simulink subsystem "Find_U_And_Powers"  (R2023b)
settings: Solver=VariableStepAuto  StartTime=0.0  StopTime=10.0  RelTol=1e-3
undefined symbols (not defined in the file): Spline_Num_Samples
settings Model: Creator=FIRSTMentor  LastModifiedBy=FIRSTMentor

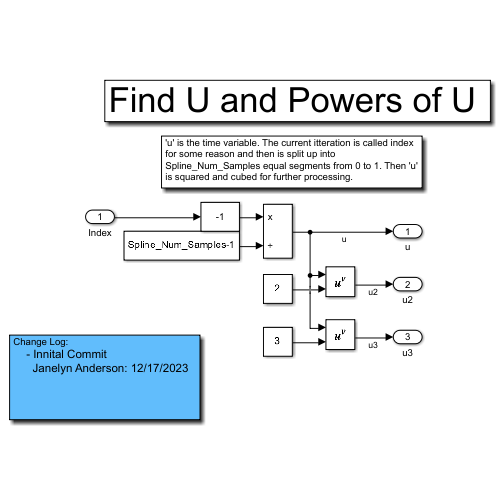
[thumbnail: Simulink's stored preview of the top-level diagram]
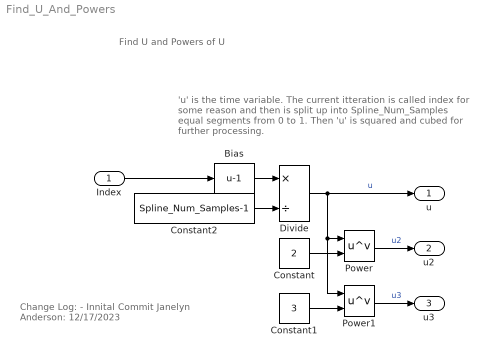
== system Find_U_And_Powers ==
  note: Change Log:
      | - Innital Commit
      | Janelyn Anderson: 12/17/2023
  note: Find U and Powers of U
  note: 'u' is the time variable. The current itteration is called index for some reason and then is split up into Spline_Num_Samples equal segments from 0 to 1. Then 'u' is squared and cubed for further processing.
  Index : Inport
  Bias : Bias  Bias=-1  SaturateOnIntegerOverflow=off
  Constant : Constant  Value=2
  Constant1 : Constant  Value=3
  Constant2 : Constant  Value=Spline_Num_Samples-1
  Divide : Product  Inputs=*/
  Power : Math  Operator=pow
  Power1 : Math  Operator=pow
  u : Outport
  u2 : Outport  Port=2
  u3 : Outport  Port=3
  wires:
  Power1/1 -> u3/1  "u3"
  Constant2/1 -> Divide/2
  Constant/1 -> Power/2
  Index/1 -> Bias/1
  Constant1/1 -> Power1/2
  Bias/1 -> Divide/1
  Power/1 -> u2/1  "u2"
  Divide/1 -> u/1, Power1/1, Power/1  "u"
